simulink model "motor_position_lqr_multibody"  (R2022b)
settings: Solver=ode15s  StartTime=0.0  StopTime=stopTime  MaxStep=0.01  RelTol=1e-8  AbsTol=1e-10
model workspace (MAT data in the model file):
  J = 0.01
  K = [1 1 1]
  K_e = 0.01
  Ki = 0
  L = 0.5
  Nbar = 1
  R_m = 1
  b = 0.1
  disturbanceTime = 3
  loadTorque = 0
  r = 1
  stopTime = 5
  umax = inf
  voltageDisturbance = 0
undefined symbols (not defined in the file or in its folder): X, Y, Z
libraries: sm_lib x6, nesl_utility x4
settings Model: Creator=shark  LastModifiedBy=shark

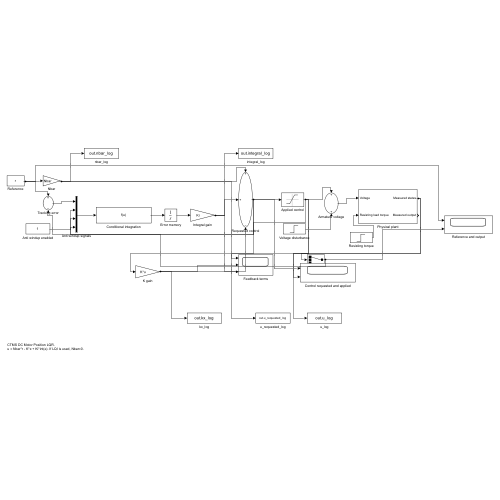
[thumbnail: Simulink's stored preview of the top-level diagram]
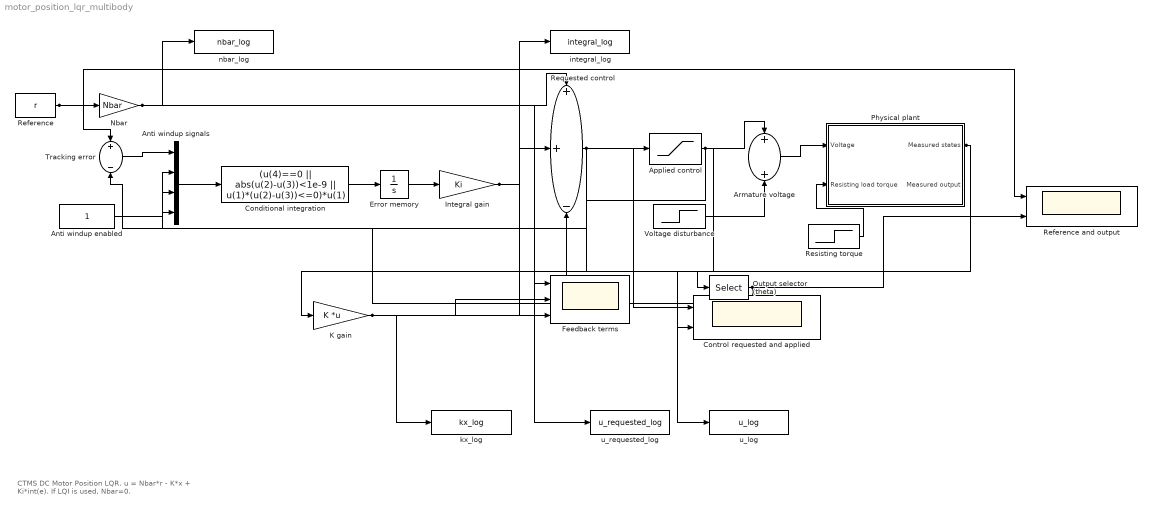
== system motor_position_lqr_multibody ==
  note: CTMS DC Motor Position LQR.
      | u = Nbar*r - K*x + Ki*int(e). If LQI is used, Nbar=0.
  Anti windup enabled : Constant
  Anti windup signals : Mux
  Applied control : Saturate  UpperLimit=umax  LowerLimit=-umax
  Armature voltage : Sum
  Conditional integration : Fcn  Expr=(u(4)==0 || abs(u(2)-u(3))<1e-9 || u(1)*(u(2)-u(3))<=0)*u(1)
  Control requested and applied : Scope  NumInputPorts=2
  Error memory : Integrator
  Feedback terms : Scope  NumInputPorts=3
  Integral gain : Gain  Gain=Ki
  K gain : Gain  Gain=K  Multiplication=Matrix(K*u)
  Nbar : Gain  Gain=Nbar
  Output selector (theta) : Selector  InputPortWidth=3  IndexOptions=Index vector (dialog)  Indices=1  OutputSizes=1
  Physical plant : Subsystem
  Reference : Constant  Value=r
  Reference and output : Scope  NumInputPorts=2
  Requested control : Sum  Inputs=++-
  Resisting torque : Step  Time=disturbanceTime  After=loadTorque  SampleTime=0
  Tracking error : Sum  Inputs=+-
  Voltage disturbance : Step  Time=disturbanceTime  After=voltageDisturbance  SampleTime=0
  integral_log : ToWorkspace  VariableName=integral_log  SaveFormat=Timeseries  SampleTime=-1
  kx_log : ToWorkspace  VariableName=kx_log  SaveFormat=Timeseries  SampleTime=-1
  nbar_log : ToWorkspace  VariableName=nbar_log  SaveFormat=Timeseries  SampleTime=-1
  u_log : ToWorkspace  VariableName=u_log  SaveFormat=Timeseries  SampleTime=-1
  u_requested_log : ToWorkspace  VariableName=u_requested_log  SaveFormat=Timeseries  SampleTime=-1
  wires:
  Reference/1 -> Nbar/1, Tracking error/1, Reference and output/1
  Physical plant/1(Measured states) -> Output selector (theta)/1, K gain/1
  Output selector (theta)/1 -> Tracking error/2, Reference and output/2
  Tracking error/1 -> Anti windup signals/1
  Requested control/1 -> Anti windup signals/2, Applied control/1, Control requested and applied/1, u_requested_log/1
  Applied control/1 -> Anti windup signals/3, Armature voltage/1, Control requested and applied/2, u_log/1
  Anti windup enabled/1 -> Anti windup signals/4
  Anti windup signals/1 -> Conditional integration/1
  Conditional integration/1 -> Error memory/1
  Error memory/1 -> Integral gain/1
  Nbar/1 -> Requested control/1, Feedback terms/1, nbar_log/1
  Integral gain/1 -> Requested control/2, Feedback terms/3, integral_log/1
  K gain/1 -> Requested control/3, Feedback terms/2, kx_log/1
  Voltage disturbance/1 -> Armature voltage/2
  Armature voltage/1 -> Physical plant/1(Voltage)
  Resisting torque/1 -> Physical plant/2(Resisting load torque)

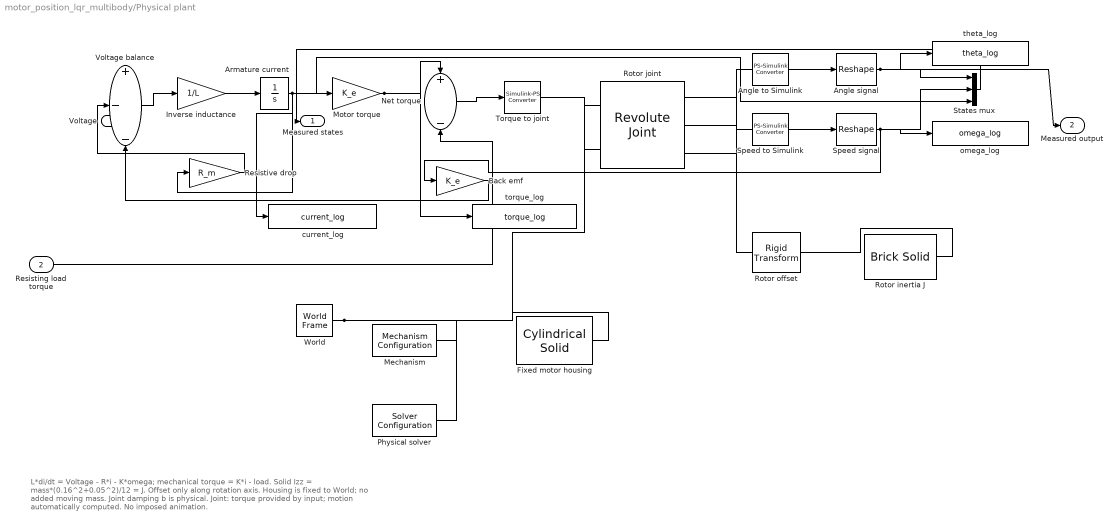
== system motor_position_lqr_multibody/Physical plant ==
  note: L*di/dt = Voltage - R*i - K*omega; mechanical torque = K*i - load.
      | Solid Izz = mass*(0.16^2+0.05^2)/12 = J. Offset only along rotation axis.
      | Housing is fixed to World; no added moving mass. Joint damping b is physical.
      | Joint: torque provided by input; motion automatically computed. No imposed animation.
  Voltage : Inport
  Resisting load torque : Inport  Port=2
  Angle signal : Reshape
  Angle to Simulink : nesl_utility/PS-Simulink Converter  PhysicalDomain=network_engine_domain  SubClassName=ps_output  LeftPortType=input  RightPortType=output  PseudoPeriodic=off  Frequencies=[]  VectorFormat=inherit  Unit=rad  AffineConversion=off
  Armature current : Integrator
  Back emf : Gain  Gain=K_e
  Fixed motor housing : sm_lib/Body Elements/Cylindrical Solid  GraphicAmbientColor=[0.15 0.15 0.15 1.0]  BasedOnType=Mass  CenterOfMass=[0 0 0]  CenterOfMassUnits=m  GraphicDiffuseColor=[0.16 0.34 0.6]  CylinderLength=.07  CylinderLengthUnits=m  CylinderRadius=.1  CylinderRadiusUnits=m  Density=1000  DensityUnits=kg/m^3  DoExposeReferenceFrame=on  GraphicEmissiveColor=[0.0 0.0 0.0 1.0]  ExportEntireGeometry=off  SerializedFrames=<Frames/>  MarkerShape=Sphere  MarkerSize=10  GraphicType=FromGeometry  InertiaType=CalculateFromGeometry  Mass=1  MassUnits=kg  MomentsOfInertia=[1 1 1]  MomentsOfInertiaUnits=kg*m^2  GraphicOpacity=1.0  ProductsOfInertia=[0 0 0]  ProductsOfInertiaUnits=kg*m^2  GraphicShininess=75  GraphicSpecularColor=[0.5 0.5 0.5 1.0]  GraphicVisPropType=SimpleVisualProperties
  Inverse inductance : Gain  Gain=1/L
  Mechanism : sm_lib/Utilities/Mechanism Configuration  UniformGravity=Constant  GravityVector=[0 0 0]  GravityUnits=m/s^2  LinearizationDelta=0.001  JointModeTransitionNonlinearIterations=2
  Motor torque : Gain  Gain=K_e
  Net torque : Sum  Inputs=+-
  Physical solver : nesl_utility/Solver Configuration  PhysicalDomain=network_engine_domain  SubClassName=solver  LeftPortType=input  RightPortType=generic  Tones=[]  Harmonics=[]  SimulateNoise=off  Profile=off  UseLocalSampling=off  EnableSwitchedLinearOptims=on  FrequencyDomain=off  UseCCode=off  RelTol=0.001  AbsTol=0.001  MinStep=1e-09  ToWorkspace=off  RevertToSquareIcSolve=off  NumHomotopyIterations=100  PhasorMode=off  PhasorModeNumHarmonics=1  ConsistencySolver=NEWTON_XTOL_AFTER_FTOL  IndexReductionMethod=DerivativeReplacement  DoDC=off  ResidualTolerance=1e-09  ConsistencyTolSource=GLOBAL  ConsistencyAbsTol=0.001  ConsistencyRelTol=0.001  ConsistencyTolFactor=0.001  UseLocalSolver=off  LocalSolverChoice=NE_BACKWARD_EULER_ADVANCER  ResolveIndetEquations=on  FunctionEvalNumThread=1  LocalSolverSampleTime=0.001  DoFixedCost=off  MaxNonlinIter=3  MaxModeIter=2  ComputeImpulses=off  ImpulseIterations=2  LinearAlgebra=auto  LinearAlgebraNumThread=0  EquationFormulation=NE_TIME_EF  DelaysMemoryBudget=1024  AutomaticFiltering=on  FilteringTimeConstant=0.001  PartitionStorageMethod=AS_NEEDED  PartitionMemoryBudget=1024  PartitionMethod=ROBUST
  Resistive drop : Gain  Gain=R_m
  Rotor inertia J : sm_lib/Body Elements/Brick Solid  GraphicAmbientColor=[0.15 0.15 0.15 1.0]  BasedOnType=Mass  BrickDimensions=[0.16 0.05 0.025]  BrickDimensionUnits=m  CenterOfMass=[0 0 0]  CenterOfMassUnits=m  GraphicDiffuseColor=[0.9 0.32 0.12]  Density=1000  DensityUnits=kg/m^3  DoExposeReferenceFrame=on  GraphicEmissiveColor=[0.0 0.0 0.0 1.0]  ExportEntireGeometry=off  SerializedFrames=<Frames/>  MarkerShape=Sphere  MarkerSize=10  GraphicType=FromGeometry  InertiaType=CalculateFromGeometry  Mass=12*J/(0.16^2+0.05^2)  MassUnits=kg  MomentsOfInertia=[1 1 1]  MomentsOfInertiaUnits=kg*m^2  GraphicOpacity=1.0  ProductsOfInertia=[0 0 0]  ProductsOfInertiaUnits=kg*m^2  GraphicShininess=75  GraphicSpecularColor=[0.5 0.5 0.5 1.0]  GraphicVisPropType=SimpleVisualProperties
  Rotor joint : sm_lib/Joints/Revolute Joint  JointMode=Normal  SenseConstraintForce=off  SenseConstraintForceX=off  SenseConstraintForceY=off  SenseConstraintForceZ=off  SenseConstraintTorque=off  SenseConstraintTorqueX=off  SenseConstraintTorqueY=off  SenseConstraintTorqueZ=off  SenseTotalForce=off  SenseTotalForceX=off  SenseTotalForceY=off  SenseTotalForceZ=off  SenseTotalTorque=off  SenseTotalTorqueX=off  SenseTotalTorqueY=off  SenseTotalTorqueZ=off  CompositeWrenchDir=FollowerOnBase  CompositeWrenchFrame=BaseFrame  EquilibriumPosition=0  EquilibriumPositionUnits=deg  SpringStiffness=0  SpringStiffnessUnits=N*m/deg  DampingCoefficient=b  DampingCoefficientUnits=N*m/(rad/s)  TorqueActuationMode=InputTorque  MotionActuationMode=ComputedMotion  SensePosition=on  SenseVelocity=on  SenseAcceleration=off  SenseTorqueForce=off  SenseLowerLimitTorqueForce=off  SenseUpperLimitTorqueForce=off  LowerLimitSpecify=off  LowerLimitBound=-90  LowerLimitBoundUnits=deg  LowerLimitStiffness=1e4  LowerLimitStiffnessUnits=N*m/deg  LowerLimitDamping=10  LowerLimitDampingUnits=N*m/(deg/s)  LowerLimitTransitionRegionWidth=0.1  LowerLimitTransitionRegionWidthUnits=deg  UpperLimitSpecify=off  UpperLimitBound=90  UpperLimitBoundUnits=deg  UpperLimitStiffness=1e4  UpperLimitStiffnessUnits=N*m/deg  UpperLimitDamping=10  UpperLimitDampingUnits=N*m/(deg/s)  UpperLimitTransitionRegionWidth=0.1  UpperLimitTransitionRegionWidthUnits=deg  PositionTargetSpecify=on  PositionTargetPriority=High  PositionTargetValue=0  PositionTargetValueUnits=deg  VelocityTargetSpecify=on  VelocityTargetPriority=High  VelocityTargetValue=0  VelocityTargetValueUnits=deg/s
  Rotor offset : sm_lib/Frames and Transforms/Rigid Transform  TranslationMethod=Cartesian  TranslationStandardOffset=0  TranslationLengthUnit=m  TranslationStandardAxis=+Z  TranslationCartesianOffset=[0 0 0.06]  TranslationROffset=0  TranslationROffsetUnits=m  TranslationZOffset=0  TranslationZOffsetUnits=m  TranslationThetaOffset=0  TranslationThetaOffsetUnits=deg  RotationMethod=None  RotationAngleUnits=deg  RotationStandardAxis=+Z  RotationAngle=0.0  RotationArbitraryAxis=[0 0 1]  FollAlignAxisA=+X  BaseAlignAxisA=+Y  FollAlignAxisB=+Y  BaseAlignAxisB=+Z  RotationSequenceAxes=FollowerAxes  RotationSequence=XYX  RotationSequenceAngles=[0 0 0]  RotationSequenceAnglesUnits=deg  RotationMatrix=[1 0 0; 0 1 0; 0 0 1]  Quaternion=[1 0 0 0]
  Speed signal : Reshape
  Speed to Simulink : nesl_utility/PS-Simulink Converter  PhysicalDomain=network_engine_domain  SubClassName=ps_output  LeftPortType=input  RightPortType=output  PseudoPeriodic=off  Frequencies=[]  VectorFormat=inherit  Unit=rad/s  AffineConversion=off
  States mux : Mux  Inputs=3
  Torque to joint : nesl_utility/Simulink-PS Converter  PhysicalDomain=network_engine_domain  SubClassName=ps_input  LeftPortType=input  RightPortType=output  PseudoPeriodic=off  Frequencies=[]  NoiseDistribution=none  NoiseParameters=[]  Unit=N*m  AffineConversion=off  FilteringAndDerivatives=provide  SimscapeFilterOrder=1  InputFilterTimeConstant=0.001  UdotUserProvided=0
  Voltage balance : Sum  Inputs=+--
  World : sm_lib/Frames and Transforms/World Frame
  current_log : ToWorkspace  VariableName=current_log  SaveFormat=Timeseries  SampleTime=-1
  omega_log : ToWorkspace  VariableName=omega_log  SaveFormat=Timeseries  SampleTime=-1
  theta_log : ToWorkspace  VariableName=theta_log  SaveFormat=Timeseries  SampleTime=-1
  torque_log : ToWorkspace  VariableName=torque_log  SaveFormat=Timeseries  SampleTime=-1
  Measured states : Outport
  Measured output : Outport  Port=2
  wires:
  Voltage/1 -> Voltage balance/1
  Resistive drop/1 -> Voltage balance/2
  Back emf/1 -> Voltage balance/3
  Voltage balance/1 -> Inverse inductance/1
  Inverse inductance/1 -> Armature current/1
  Armature current/1 -> Resistive drop/1, Motor torque/1, States mux/3, current_log/1
  Motor torque/1 -> Net torque/1, torque_log/1
  Resisting load torque/1 -> Net torque/2
  Net torque/1 -> Torque to joint/1
  Angle to Simulink/1 -> Angle signal/1
  Speed to Simulink/1 -> Speed signal/1
  Speed signal/1 -> Back emf/1, States mux/2, omega_log/1
  Angle signal/1 -> States mux/1, Measured output/1, theta_log/1
  States mux/1 -> Measured states/1
  connections:
  Rotor joint/LConn1 -- World/RConn1 -- Fixed motor housing/RConn1 -- Mechanism/RConn1 -- Physical solver/RConn1
  Torque to joint/RConn1 -- Rotor joint/LConn2
  Rotor joint/RConn1 -- Rotor offset/LConn1
  Rotor offset/RConn1 -- Rotor inertia J/RConn1
  Rotor joint/RConn2 -- Angle to Simulink/LConn1
  Rotor joint/RConn3 -- Speed to Simulink/LConn1
